simulink model "COSTEP_Exergy"  (R2024b)
settings: Solver=FixedStepAuto  StartTime=0.0  StopTime=25  FixedStep=1/3600  RelTol=1e-3
model workspace (MAT data in the model file):
  AD : Simulink.Parameter (value not decoded)
  AG : Simulink.Parameter (value not decoded)
  AH : Simulink.Parameter (value not decoded)
  AV : Simulink.Parameter (value not decoded)
  AVP : Simulink.Parameter (value not decoded)
  BCHL : Simulink.Parameter (value not decoded)
  BCHV : Simulink.Parameter (value not decoded)
  BD : Simulink.Parameter (value not decoded)
  BDIST : Simulink.Parameter (value not decoded)
  BG : Simulink.Parameter (value not decoded)
  BH : Simulink.Parameter (value not decoded)
  BVP : Simulink.Parameter (value not decoded)
  CD : Simulink.Parameter (value not decoded)
  CDIST : Simulink.Parameter (value not decoded)
  CG : Simulink.Parameter (value not decoded)
  CH : Simulink.Parameter (value not decoded)
  CVP : Simulink.Parameter (value not decoded)
  DDIST : Simulink.Parameter (value not decoded)
  DIST_CONST : Simulink.Parameter (value not decoded)
  ISV : Simulink.Parameter (value not decoded)
  TLAST : Simulink.Parameter (value not decoded)
  TNEXT : Simulink.Parameter (value not decoded)
  XMW : Simulink.Parameter (value not decoded)
  XNS : Simulink.Parameter (value not decoded)
  XNS2 : Simulink.Parameter (value not decoded)
  XNS3 : Simulink.Parameter (value not decoded)
  XNSADD : Simulink.Parameter (value not decoded)
  XNSE : Simulink.Parameter (value not decoded)
symbols that are objects in the model workspace (value not decoded): AD, AG, AH, AV, AVP, BD, BG, BH, BVP, CD, CG, CH, CVP, XMW, XNS, XNS2, XNS3, XNSE
undefined symbols (not defined in the file or in its folder): magnitude, msgbox, SETPT, XMEAS, XMV
libraries: mylib x403, dspindex x31
(part 12 of 13)

== system COSTEP_Exergy/Stream Measurements/Subsystem6/E feed stream/Composition measurement mol%/Subsystem/Subsystem ==
  XST : Inport
  Constant : Constant  Value=100
  Multiport Selector : dspindex/Multiport Selector  rowsOrCols=Rows  idxCellArray={ 5,6}  idxErrMode=Clip Index
  Product : Product
  Product1 : Product
  "XCMPE " : Outport  VectorParamsAs1DForOutWhenUnconnected=off
  "XCMPF " : Outport  Port=2  VectorParamsAs1DForOutWhenUnconnected=off
  wires:
  Multiport Selector/1 -> Product/1
  Constant/1 -> Product/2, Product1/2
  XST/1 -> Multiport Selector/1
  Multiport Selector/2 -> Product1/1
  Product/1 -> "XCMPE "/1
  Product1/1 -> "XCMPF "/1

== system COSTEP_Exergy/Stream Measurements/Subsystem6/Product stream/Composition measurement mol%/Subsystem/Subsystem ==
  XST : Inport
  Constant : Constant  Value=100
  Multiport Selector : dspindex/Multiport Selector  rowsOrCols=Rows  idxCellArray={ 1,2,3}  idxErrMode=Clip Index
  Product : Product
  Product1 : Product
  Product2 : Product
  XCMPA : Outport  VectorParamsAs1DForOutWhenUnconnected=off
  XCMPB : Outport  Port=2  VectorParamsAs1DForOutWhenUnconnected=off
  XCMPC : Outport  Port=3  VectorParamsAs1DForOutWhenUnconnected=off
  wires:
  Multiport Selector/1 -> Product/1
  Multiport Selector/3 -> Product2/1
  Constant/1 -> Product2/2, Product/2, Product1/2
  XST/1 -> Multiport Selector/1
  Multiport Selector/2 -> Product1/1
  Product/1 -> XCMPA/1
  Product1/1 -> XCMPB/1
  Product2/1 -> XCMPC/1

== system COSTEP_Exergy/Stream Measurements/Subsystem6/Product stream/Composition measurement mol%/Subsystem1/Subsystem ==
  XST : Inport
  Constant : Constant  Value=100
  Multiport Selector : dspindex/Multiport Selector  rowsOrCols=Rows  idxCellArray={4,5,6,7,8}  idxErrMode=Clip Index
  "XCMPD " : Product
  XCMPE : Product
  XCMPF : Product
  "XCMPG " : Product
  XCMPH : Product
  XCMPD : Outport  VectorParamsAs1DForOutWhenUnconnected=off
  "XCMPE " : Outport  Port=2  VectorParamsAs1DForOutWhenUnconnected=off
  "XCMPF " : Outport  Port=3  VectorParamsAs1DForOutWhenUnconnected=off
  XCMPG : Outport  Port=4  VectorParamsAs1DForOutWhenUnconnected=off
  "XCMPH " : Outport  Port=5  VectorParamsAs1DForOutWhenUnconnected=off
  wires:
  Constant/1 -> XCMPE/2, "XCMPG "/2, XCMPH/2, XCMPF/2, "XCMPD "/2
  Multiport Selector/1 -> "XCMPD "/1
  "XCMPD "/1 -> XCMPD/1  "XCMPD"
  Multiport Selector/5 -> XCMPH/1
  XCMPF/1 -> "XCMPF "/1  "XCMPF"
  XST/1 -> Multiport Selector/1
  Multiport Selector/4 -> "XCMPG "/1
  Multiport Selector/2 -> XCMPE/1
  Multiport Selector/3 -> XCMPF/1
  XCMPE/1 -> "XCMPE "/1  "XCMPE"
  XCMPH/1 -> "XCMPH "/1  "XCMPH"
  "XCMPG "/1 -> XCMPG/1  "XCMPG"

== system COSTEP_Exergy/Stream Measurements/Subsystem6/Reactor feed stream/Composition measurement mol%/Subsystem/Subsystem ==
  XST : Inport
  Constant : Constant  Value=100
  Multiport Selector : dspindex/Multiport Selector  rowsOrCols=Rows  idxCellArray={7,8}  idxErrMode=Clip Index
  Product6 : Product
  Product7 : Product
  XCMPG : Outport  VectorParamsAs1DForOutWhenUnconnected=off
  "XCMPH " : Outport  Port=2  VectorParamsAs1DForOutWhenUnconnected=off
  wires:
  Multiport Selector/2 -> Product7/1
  Multiport Selector/1 -> Product6/1
  Constant/1 -> Product6/2, Product7/2
  XST/1 -> Multiport Selector/1
  Product6/1 -> XCMPG/1
  Product7/1 -> "XCMPH "/1

== system COSTEP_Exergy/Stream Measurements/Subsystem6/Reactor product stream/Composition measurement mol%/Subsystem/Subsystem ==
  XST : Inport
  Constant : Constant  Value=100
  Multiport Selector : dspindex/Multiport Selector  rowsOrCols=Rows  idxCellArray={ 1,2,3,4,5,6,7,8}  idxErrMode=Clip Index
  Product{,1..7} (8 alike) : Product
  XCMPA : Outport  VectorParamsAs1DForOutWhenUnconnected=off
  XCMPB : Outport  Port=2  VectorParamsAs1DForOutWhenUnconnected=off
  XCMPC : Outport  Port=3  VectorParamsAs1DForOutWhenUnconnected=off
  XCMPD : Outport  Port=4  VectorParamsAs1DForOutWhenUnconnected=off
  "XCMPE " : Outport  Port=5  VectorParamsAs1DForOutWhenUnconnected=off
  "XCMPF " : Outport  Port=6  VectorParamsAs1DForOutWhenUnconnected=off
  XCMPG : Outport  Port=7  VectorParamsAs1DForOutWhenUnconnected=off
  "XCMPH " : Outport  Port=8  VectorParamsAs1DForOutWhenUnconnected=off
  wires:
  Multiport Selector/6 -> Product5/1
  Multiport Selector/8 -> Product7/1
  Multiport Selector/5 -> Product4/1
  Multiport Selector/7 -> Product6/1
  Multiport Selector/1 -> Product/1
  Multiport Selector/3 -> Product2/1
  Constant/1 -> Product/2, Product1/2, Product2/2, Product3/2, Product4/2, Product5/2, Product7/2, Product6/2
  Multiport Selector/4 -> Product3/1
  XST/1 -> Multiport Selector/1
  Multiport Selector/2 -> Product1/1
  Product/1 -> XCMPA/1
  Product1/1 -> XCMPB/1
  Product2/1 -> XCMPC/1
  Product3/1 -> XCMPD/1
  Product4/1 -> "XCMPE "/1
  Product5/1 -> "XCMPF "/1
  Product6/1 -> XCMPG/1
  Product7/1 -> "XCMPH "/1

== system COSTEP_Exergy/Stream Measurements/Subsystem6/Separator product stream/Composition measurement mol%/Subsystem/Subsystem ==
  XST : Inport
  Constant : Constant  Value=100
  Multiport Selector : dspindex/Multiport Selector  rowsOrCols=Rows  idxCellArray={ 1,2,3,4,5,6,7,8}  idxErrMode=Clip Index
  Product{,1..7} (8 alike) : Product
  XCMPA : Outport  VectorParamsAs1DForOutWhenUnconnected=off
  XCMPB : Outport  Port=2  VectorParamsAs1DForOutWhenUnconnected=off
  XCMPC : Outport  Port=3  VectorParamsAs1DForOutWhenUnconnected=off
  XCMPD : Outport  Port=4  VectorParamsAs1DForOutWhenUnconnected=off
  "XCMPE " : Outport  Port=5  VectorParamsAs1DForOutWhenUnconnected=off
  "XCMPF " : Outport  Port=6  VectorParamsAs1DForOutWhenUnconnected=off
  XCMPG : Outport  Port=7  VectorParamsAs1DForOutWhenUnconnected=off
  "XCMPH " : Outport  Port=8  VectorParamsAs1DForOutWhenUnconnected=off
  wires:
  Multiport Selector/6 -> Product5/1
  Multiport Selector/8 -> Product7/1
  Multiport Selector/5 -> Product4/1
  Multiport Selector/7 -> Product6/1
  Multiport Selector/1 -> Product/1
  Multiport Selector/3 -> Product2/1
  Constant/1 -> Product/2, Product1/2, Product2/2, Product3/2, Product4/2, Product5/2, Product7/2, Product6/2
  Multiport Selector/4 -> Product3/1
  XST/1 -> Multiport Selector/1
  Multiport Selector/2 -> Product1/1
  Product/1 -> XCMPA/1
  Product1/1 -> XCMPB/1
  Product2/1 -> XCMPC/1
  Product3/1 -> XCMPD/1
  Product4/1 -> "XCMPE "/1
  Product5/1 -> "XCMPF "/1
  Product6/1 -> XCMPG/1
  Product7/1 -> "XCMPH "/1

== system COSTEP_Exergy/Stream Measurements/Subsystem6/Separator product stream/Flow measurement in kg//h/Subsystem/XMWS Molecular weight of Stream lb//lb-mol ==
  XST : Inport
  Product : Product
  Sum of Elements : Sum  Inputs=+
  "XMW(I) Molecular weight of components lb/lb-mol " : Constant  Value=XMW
  XMWS : Outport  VectorParamsAs1DForOutWhenUnconnected=off
  wires:
  Sum of Elements/1 -> XMWS/1
  Product/1 -> Sum of Elements/1
  XST/1 -> Product/1
  "XMW(I) Molecular weight of components lb/lb-mol "/1 -> Product/2

== system COSTEP_Exergy/Stream Measurements/Subsystem6/Separator product stream/Flow measurement in kg//h/Subsystem1/XMWS Molecular weight of Stream lb//lb-mol ==
  XST : Inport
  Product : Product
  Sum of Elements : Sum  Inputs=+
  "XMW(I) Molecular weight of components lb/lb-mol " : Constant  Value=XMW
  XMWS : Outport  VectorParamsAs1DForOutWhenUnconnected=off
  wires:
  Sum of Elements/1 -> XMWS/1
  Product/1 -> Sum of Elements/1
  XST/1 -> Product/1
  "XMW(I) Molecular weight of components lb/lb-mol "/1 -> Product/2

== system COSTEP_Exergy/Stream Measurements/Subsystem6/Separator recycle stream (after compressor)/Composition measurement mol%/Subsystem/Subsystem ==
  XST : Inport
  Constant : Constant  Value=100
  Multiport Selector : dspindex/Multiport Selector  rowsOrCols=Rows  idxCellArray={ 1,2,3,4,5,6,7,8}  idxErrMode=Clip Index
  Product{,1..7} (8 alike) : Product
  XCMPA : Outport  VectorParamsAs1DForOutWhenUnconnected=off
  XCMPB : Outport  Port=2  VectorParamsAs1DForOutWhenUnconnected=off
  XCMPC : Outport  Port=3  VectorParamsAs1DForOutWhenUnconnected=off
  XCMPD : Outport  Port=4  VectorParamsAs1DForOutWhenUnconnected=off
  "XCMPE " : Outport  Port=5  VectorParamsAs1DForOutWhenUnconnected=off
  "XCMPF " : Outport  Port=6  VectorParamsAs1DForOutWhenUnconnected=off
  XCMPG : Outport  Port=7  VectorParamsAs1DForOutWhenUnconnected=off
  "XCMPH " : Outport  Port=8  VectorParamsAs1DForOutWhenUnconnected=off
  wires:
  Multiport Selector/6 -> Product5/1
  Multiport Selector/8 -> Product7/1
  Multiport Selector/5 -> Product4/1
  Multiport Selector/7 -> Product6/1
  Multiport Selector/1 -> Product/1
  Multiport Selector/3 -> Product2/1
  Constant/1 -> Product/2, Product1/2, Product2/2, Product3/2, Product4/2, Product5/2, Product7/2, Product6/2
  Multiport Selector/4 -> Product3/1
  XST/1 -> Multiport Selector/1
  Multiport Selector/2 -> Product1/1
  Product/1 -> XCMPA/1
  Product1/1 -> XCMPB/1
  Product2/1 -> XCMPC/1
  Product3/1 -> XCMPD/1
  Product4/1 -> "XCMPE "/1
  Product5/1 -> "XCMPF "/1
  Product6/1 -> XCMPG/1
  Product7/1 -> "XCMPH "/1

== system COSTEP_Exergy/Stream Measurements/Subsystem6/Separator recycle stream (before compressor)/Composition measurement mol%/Subsystem/Subsystem ==
  XST : Inport
  Constant : Constant  Value=100
  Multiport Selector : dspindex/Multiport Selector  rowsOrCols=Rows  idxCellArray={ 1,2,3,4,5,6,7,8}  idxErrMode=Clip Index
  Product{,1..7} (8 alike) : Product
  XCMPA : Outport  VectorParamsAs1DForOutWhenUnconnected=off
  XCMPB : Outport  Port=2  VectorParamsAs1DForOutWhenUnconnected=off
  XCMPC : Outport  Port=3  VectorParamsAs1DForOutWhenUnconnected=off
  XCMPD : Outport  Port=4  VectorParamsAs1DForOutWhenUnconnected=off
  "XCMPE " : Outport  Port=5  VectorParamsAs1DForOutWhenUnconnected=off
  "XCMPF " : Outport  Port=6  VectorParamsAs1DForOutWhenUnconnected=off
  XCMPG : Outport  Port=7  VectorParamsAs1DForOutWhenUnconnected=off
  "XCMPH " : Outport  Port=8  VectorParamsAs1DForOutWhenUnconnected=off
  wires:
  Multiport Selector/6 -> Product5/1
  Multiport Selector/8 -> Product7/1
  Multiport Selector/5 -> Product4/1
  Multiport Selector/7 -> Product6/1
  Multiport Selector/1 -> Product/1
  Multiport Selector/3 -> Product2/1
  Constant/1 -> Product/2, Product1/2, Product2/2, Product3/2, Product4/2, Product5/2, Product7/2, Product6/2
  Multiport Selector/4 -> Product3/1
  XST/1 -> Multiport Selector/1
  Multiport Selector/2 -> Product1/1
  Product/1 -> XCMPA/1
  Product1/1 -> XCMPB/1
  Product2/1 -> XCMPC/1
  Product3/1 -> XCMPD/1
  Product4/1 -> "XCMPE "/1
  Product5/1 -> "XCMPF "/1
  Product6/1 -> XCMPG/1
  Product7/1 -> "XCMPH "/1

== system COSTEP_Exergy/Stream Measurements/Subsystem6/Separator underflow stream/Composition measurement mol%/Subsystem/Subsystem ==
  XST : Inport
  Constant : Constant  Value=100
  Multiport Selector : dspindex/Multiport Selector  rowsOrCols=Rows  idxCellArray={ 4,5,6,7,8}  idxErrMode=Clip Index
  Product{3..7} (5 alike) : Product
  XCMPD : Outport  VectorParamsAs1DForOutWhenUnconnected=off
  "XCMPE " : Outport  Port=2  VectorParamsAs1DForOutWhenUnconnected=off
  "XCMPF " : Outport  Port=3  VectorParamsAs1DForOutWhenUnconnected=off
  XCMPG : Outport  Port=4  VectorParamsAs1DForOutWhenUnconnected=off
  "XCMPH " : Outport  Port=5  VectorParamsAs1DForOutWhenUnconnected=off
  wires:
  Constant/1 -> Product3/2, Product4/2, Product5/2, Product7/2, Product6/2
  XST/1 -> Multiport Selector/1
  Product3/1 -> XCMPD/1
  Product4/1 -> "XCMPE "/1
  Product5/1 -> "XCMPF "/1
  Product6/1 -> XCMPG/1
  Product7/1 -> "XCMPH "/1
  Multiport Selector/1 -> Product3/1
  Multiport Selector/2 -> Product4/1
  Multiport Selector/3 -> Product5/1
  Multiport Selector/4 -> Product6/1
  Multiport Selector/5 -> Product7/1

== system COSTEP_Exergy/Stream Measurements/Subsystem6/Stripper recycle stream/Composition measurement mol%/Subsystem/Subsystem ==
  XST : Inport
  Constant : Constant  Value=100
  Multiport Selector : dspindex/Multiport Selector  rowsOrCols=Rows  idxCellArray={ 1,2,3,4,5,6,7,8}  idxErrMode=Clip Index
  Product{,1..7} (8 alike) : Product
  XCMPA : Outport  VectorParamsAs1DForOutWhenUnconnected=off
  XCMPB : Outport  Port=2  VectorParamsAs1DForOutWhenUnconnected=off
  XCMPC : Outport  Port=3  VectorParamsAs1DForOutWhenUnconnected=off
  XCMPD : Outport  Port=4  VectorParamsAs1DForOutWhenUnconnected=off
  "XCMPE " : Outport  Port=5  VectorParamsAs1DForOutWhenUnconnected=off
  "XCMPF " : Outport  Port=6  VectorParamsAs1DForOutWhenUnconnected=off
  XCMPG : Outport  Port=7  VectorParamsAs1DForOutWhenUnconnected=off
  "XCMPH " : Outport  Port=8  VectorParamsAs1DForOutWhenUnconnected=off
  wires:
  Multiport Selector/6 -> Product5/1
  Multiport Selector/8 -> Product7/1
  Multiport Selector/5 -> Product4/1
  Multiport Selector/7 -> Product6/1
  Multiport Selector/1 -> Product/1
  Multiport Selector/3 -> Product2/1
  Constant/1 -> Product/2, Product1/2, Product2/2, Product3/2, Product4/2, Product5/2, Product7/2, Product6/2
  Multiport Selector/4 -> Product3/1
  XST/1 -> Multiport Selector/1
  Multiport Selector/2 -> Product1/1
  Product/1 -> XCMPA/1
  Product1/1 -> XCMPB/1
  Product2/1 -> XCMPC/1
  Product3/1 -> XCMPD/1
  Product4/1 -> "XCMPE "/1
  Product5/1 -> "XCMPF "/1
  Product6/1 -> XCMPG/1
  Product7/1 -> "XCMPH "/1

== system COSTEP_Exergy/Subsystem1/Condenser cooling water/CCin/Subsystem3/Subsystem/Subsystem2 ==
  T1 : Inport
  T0 : Inport  Port=2
  A : Constant  Value=9.069
  Add1 : Sum  Inputs=+-
  Product1 : Product
  AT : Outport
  wires:
  Add1/1 -> Product1/2
  A/1 -> Product1/1
  T0/1 -> Add1/2
  T1/1 -> Add1/1
  Product1/1 -> AT/1

== system COSTEP_Exergy/Subsystem1/Condenser cooling water/CCin/Subsystem3/Subsystem1/Subsystem ==
  T1 : Inport
  T0 : Inport  Port=2
  A : Constant  Value=9.069
  Divide : Product  Inputs=*/
  Math Function : Math  Operator=log  SignedPower=on
  Product1 : Product
  AT : Outport
  wires:
  Product1/1 -> AT/1
  A/1 -> Product1/1
  T1/1 -> Divide/1
  T0/1 -> Divide/2
  Math Function/1 -> Product1/2
  Divide/1 -> Math Function/1

== system COSTEP_Exergy/Subsystem1/Condenser cooling water/CCout/Subsystem3/Subsystem/Subsystem2 ==
  T1 : Inport
  T0 : Inport  Port=2
  A : Constant  Value=9.069
  Add1 : Sum  Inputs=+-
  Product1 : Product
  AT : Outport
  wires:
  Add1/1 -> Product1/2
  A/1 -> Product1/1
  T0/1 -> Add1/2
  T1/1 -> Add1/1
  Product1/1 -> AT/1

== system COSTEP_Exergy/Subsystem1/Condenser cooling water/CCout/Subsystem3/Subsystem1/Subsystem ==
  T1 : Inport
  T0 : Inport  Port=2
  A : Constant  Value=9.069
  Divide : Product  Inputs=*/
  Math Function : Math  Operator=log  SignedPower=on
  Product1 : Product
  AT : Outport
  wires:
  Product1/1 -> AT/1
  A/1 -> Product1/1
  T1/1 -> Divide/1
  T0/1 -> Divide/2
  Math Function/1 -> Product1/2
  Divide/1 -> Math Function/1

== system COSTEP_Exergy/Subsystem1/Reactor cooling water/RCin/Subsystem3/Subsystem/Subsystem2 ==
  T1 : Inport
  T0 : Inport  Port=2
  A : Constant  Value=9.069
  Add1 : Sum  Inputs=+-
  Product1 : Product
  AT : Outport
  wires:
  Add1/1 -> Product1/2
  A/1 -> Product1/1
  T0/1 -> Add1/2
  T1/1 -> Add1/1
  Product1/1 -> AT/1

== system COSTEP_Exergy/Subsystem1/Reactor cooling water/RCin/Subsystem3/Subsystem1/Subsystem ==
  T1 : Inport
  T0 : Inport  Port=2
  A : Constant  Value=9.069
  Divide : Product  Inputs=*/
  Math Function : Math  Operator=log  SignedPower=on
  Product1 : Product
  AT : Outport
  wires:
  Product1/1 -> AT/1
  A/1 -> Product1/1
  T1/1 -> Divide/1
  T0/1 -> Divide/2
  Math Function/1 -> Product1/2
  Divide/1 -> Math Function/1

== system COSTEP_Exergy/Subsystem1/Reactor cooling water/RCout/Subsystem3/Subsystem/Subsystem2 ==
  T1 : Inport
  T0 : Inport  Port=2
  A : Constant  Value=9.069
  Add1 : Sum  Inputs=+-
  Product1 : Product
  AT : Outport
  wires:
  Add1/1 -> Product1/2
  A/1 -> Product1/1
  T0/1 -> Add1/2
  T1/1 -> Add1/1
  Product1/1 -> AT/1

== system COSTEP_Exergy/Subsystem1/Reactor cooling water/RCout/Subsystem3/Subsystem1/Subsystem ==
  T1 : Inport
  T0 : Inport  Port=2
  A : Constant  Value=9.069
  Divide : Product  Inputs=*/
  Math Function : Math  Operator=log  SignedPower=on
  Product1 : Product
  AT : Outport
  wires:
  Product1/1 -> AT/1
  A/1 -> Product1/1
  T1/1 -> Divide/1
  T0/1 -> Divide/2
  Math Function/1 -> Product1/2
  Divide/1 -> Math Function/1

== system COSTEP_Exergy/Control Mode/Braatz/ 10/CONTROL 6/P Control Velocity form/Pressure limits/If Action Subsystem ==
  In1 : Inport
  Action Port : ActionPort  ActionPortLabel=if(u1 >= 2950)
  Out1 : Outport  VectorParamsAs1DForOutWhenUnconnected=off
  wires:
  In1/1 -> Out1/1

== system COSTEP_Exergy/Control Mode/Braatz/ 10/CONTROL 6/P Control Velocity form/Pressure limits/If Action Subsystem1 ==
  In1 : Inport
  Action Port : ActionPort  ActionPortLabel=elseif(u1 <= 2300)
  Out1 : Outport  VectorParamsAs1DForOutWhenUnconnected=off
  wires:
  In1/1 -> Out1/1

== system COSTEP_Exergy/Control Mode/Braatz/ 10/CONTROL 6/P Control Velocity form/Pressure limits/If Action Subsystem2 ==
  In1 : Inport
  Action Port : ActionPort  ActionPortLabel=else
  Out1 : Outport  VectorParamsAs1DForOutWhenUnconnected=off
  wires:
  In1/1 -> Out1/1

== system COSTEP_Exergy/Random number generator/Stream Measurements SMEAS Gas analysis1/If Action Subsystem3/Subsystem/Stream 1/Subsystem/TESUB6 XMNSEA ==
  G : Inport
  Process Noise I=1-12 G New : mylib/Process Noise I=1-12 G New  SystemSampleTime=-1  VariantActivationTime=update diagram  AllowFlexibleInterface=on  Latency=0  AutoFrameSizeCalculation=off
  XNSEA : Constant  Value=0.25
  XMNSEA : Outport  VectorParamsAs1DForOutWhenUnconnected=off
  G_NEW : Outport  Port=2  VectorParamsAs1DForOutWhenUnconnected=off
  wires:
  XNSEA/1 -> Process Noise I=1-12 G New/1
  Process Noise I=1-12 G New/1 -> XMNSEA/1
  G/1 -> Process Noise I=1-12 G New/2
  Process Noise I=1-12 G New/2 -> G_NEW/1

== system COSTEP_Exergy/Random number generator/Stream Measurements SMEAS Gas analysis1/If Action Subsystem3/Subsystem/Stream 1/Subsystem/TESUB6 XMNSEB ==
  G : Inport
  Process Noise I=1-12 G New : mylib/Process Noise I=1-12 G New  SystemSampleTime=-1  VariantActivationTime=update diagram  AllowFlexibleInterface=on  Latency=0  AutoFrameSizeCalculation=off
  XNSEB : Constant  Value=0.1
  XMNSEB : Outport  VectorParamsAs1DForOutWhenUnconnected=off
  G_NEW : Outport  Port=2  VectorParamsAs1DForOutWhenUnconnected=off
  wires:
  XNSEB/1 -> Process Noise I=1-12 G New/1
  Process Noise I=1-12 G New/1 -> XMNSEB/1
  G/1 -> Process Noise I=1-12 G New/2
  Process Noise I=1-12 G New/2 -> G_NEW/1

== system COSTEP_Exergy/Random number generator/Stream Measurements SMEAS Gas analysis1/If Action Subsystem3/Subsystem/Stream 1/Subsystem/TESUB6 XMNSEC ==
  G : Inport
  Process Noise I=1-12 G New : mylib/Process Noise I=1-12 G New  SystemSampleTime=-1  VariantActivationTime=update diagram  AllowFlexibleInterface=on  Latency=0  AutoFrameSizeCalculation=off
  XNSEC : Constant  Value=0.25
  XMNSEC : Outport  VectorParamsAs1DForOutWhenUnconnected=off
  G_NEW : Outport  Port=2  VectorParamsAs1DForOutWhenUnconnected=off
  wires:
  XNSEC/1 -> Process Noise I=1-12 G New/1
  Process Noise I=1-12 G New/1 -> XMNSEC/1
  G/1 -> Process Noise I=1-12 G New/2
  Process Noise I=1-12 G New/2 -> G_NEW/1

== system COSTEP_Exergy/Random number generator/Stream Measurements SMEAS Gas analysis1/If Action Subsystem3/Subsystem/Stream 1/Subsystem/TESUB6 XMNSED ==
  G : Inport
  Process Noise I=1-12 G New : mylib/Process Noise I=1-12 G New  SystemSampleTime=-1  VariantActivationTime=update diagram  AllowFlexibleInterface=on  Latency=0  AutoFrameSizeCalculation=off
  XNSED : Constant  Value=0.1
  XMNSED : Outport  VectorParamsAs1DForOutWhenUnconnected=off
  G_NEW : Outport  Port=2  VectorParamsAs1DForOutWhenUnconnected=off
  wires:
  XNSED/1 -> Process Noise I=1-12 G New/1
  Process Noise I=1-12 G New/1 -> XMNSED/1
  G/1 -> Process Noise I=1-12 G New/2
  Process Noise I=1-12 G New/2 -> G_NEW/1

== system COSTEP_Exergy/Random number generator/Stream Measurements SMEAS Gas analysis1/If Action Subsystem3/Subsystem/Stream 1/Subsystem/TESUB6 XMNSEE ==
  G : Inport
  Process Noise I=1-12 G New : mylib/Process Noise I=1-12 G New  SystemSampleTime=-1  VariantActivationTime=update diagram  AllowFlexibleInterface=on  Latency=0  AutoFrameSizeCalculation=off
  XNSEE : Constant  Value=0.25
  XMNSEE : Outport  VectorParamsAs1DForOutWhenUnconnected=off
  G_NEW : Outport  Port=2  VectorParamsAs1DForOutWhenUnconnected=off
  wires:
  XNSEE/1 -> Process Noise I=1-12 G New/1
  Process Noise I=1-12 G New/1 -> XMNSEE/1
  G/1 -> Process Noise I=1-12 G New/2
  Process Noise I=1-12 G New/2 -> G_NEW/1

== system COSTEP_Exergy/Random number generator/Stream Measurements SMEAS Gas analysis1/If Action Subsystem3/Subsystem/Stream 1/Subsystem/TESUB6 XMNSEF ==
  G : Inport
  Process Noise I=1-12 G New : mylib/Process Noise I=1-12 G New  SystemSampleTime=-1  VariantActivationTime=update diagram  AllowFlexibleInterface=on  Latency=0  AutoFrameSizeCalculation=off
  XNSEF : Constant  Value=0.025
  XMNSEF : Outport  VectorParamsAs1DForOutWhenUnconnected=off
  G_NEW : Outport  Port=2  VectorParamsAs1DForOutWhenUnconnected=off
  wires:
  XNSEF/1 -> Process Noise I=1-12 G New/1
  Process Noise I=1-12 G New/1 -> XMNSEF/1
  G/1 -> Process Noise I=1-12 G New/2
  Process Noise I=1-12 G New/2 -> G_NEW/1

== system COSTEP_Exergy/Random number generator/Stream Measurements SMEAS Gas analysis1/If Action Subsystem3/Subsystem/Stream 1/Subsystem/TESUB6 XMNSEG ==
  G : Inport
  Process Noise I=1-12 G New : mylib/Process Noise I=1-12 G New  SystemSampleTime=-1  VariantActivationTime=update diagram  AllowFlexibleInterface=on  Latency=0  AutoFrameSizeCalculation=off
  XNSEG : Constant  Value=0.05
  XMNSEG : Outport  VectorParamsAs1DForOutWhenUnconnected=off
  G_NEW : Outport  Port=2  VectorParamsAs1DForOutWhenUnconnected=off
  wires:
  XNSEG/1 -> Process Noise I=1-12 G New/1
  Process Noise I=1-12 G New/1 -> XMNSEG/1
  G/1 -> Process Noise I=1-12 G New/2
  Process Noise I=1-12 G New/2 -> G_NEW/1

== system COSTEP_Exergy/Random number generator/Stream Measurements SMEAS Gas analysis1/If Action Subsystem3/Subsystem/Stream 1/Subsystem/TESUB6 XMNSEH ==
  G : Inport
  Process Noise I=1-12 G New : mylib/Process Noise I=1-12 G New  SystemSampleTime=-1  VariantActivationTime=update diagram  AllowFlexibleInterface=on  Latency=0  AutoFrameSizeCalculation=off
  XNSEH : Constant  Value=0.05
  XMNSEH : Outport  VectorParamsAs1DForOutWhenUnconnected=off
  G_NEW : Outport  Port=2  VectorParamsAs1DForOutWhenUnconnected=off
  wires:
  XNSEH/1 -> Process Noise I=1-12 G New/1
  Process Noise I=1-12 G New/1 -> XMNSEH/1
  G/1 -> Process Noise I=1-12 G New/2
  Process Noise I=1-12 G New/2 -> G_NEW/1

== system COSTEP_Exergy/Random number generator/Stream Measurements SMEAS Gas analysis1/If Action Subsystem3/Subsystem/Stream 13/Subsystem/TESUB6 XMNSEA ==
  G : Inport
  Process Noise I=1-12 G New : mylib/Process Noise I=1-12 G New  SystemSampleTime=-1  VariantActivationTime=update diagram  AllowFlexibleInterface=on  Latency=0  AutoFrameSizeCalculation=off
  XNSEA : Constant  Value=0.25
  XMNSEA : Outport  VectorParamsAs1DForOutWhenUnconnected=off
  G_NEW : Outport  Port=2  VectorParamsAs1DForOutWhenUnconnected=off
  wires:
  XNSEA/1 -> Process Noise I=1-12 G New/1
  Process Noise I=1-12 G New/1 -> XMNSEA/1
  G/1 -> Process Noise I=1-12 G New/2
  Process Noise I=1-12 G New/2 -> G_NEW/1

== system COSTEP_Exergy/Random number generator/Stream Measurements SMEAS Gas analysis1/If Action Subsystem3/Subsystem/Stream 13/Subsystem/TESUB6 XMNSEB ==
  G : Inport
  Process Noise I=1-12 G New : mylib/Process Noise I=1-12 G New  SystemSampleTime=-1  VariantActivationTime=update diagram  AllowFlexibleInterface=on  Latency=0  AutoFrameSizeCalculation=off
  XNSEB : Constant  Value=0.1
  XMNSEB : Outport  VectorParamsAs1DForOutWhenUnconnected=off
  G_NEW : Outport  Port=2  VectorParamsAs1DForOutWhenUnconnected=off
  wires:
  XNSEB/1 -> Process Noise I=1-12 G New/1
  Process Noise I=1-12 G New/1 -> XMNSEB/1
  G/1 -> Process Noise I=1-12 G New/2
  Process Noise I=1-12 G New/2 -> G_NEW/1

== system COSTEP_Exergy/Random number generator/Stream Measurements SMEAS Gas analysis1/If Action Subsystem3/Subsystem/Stream 13/Subsystem/TESUB6 XMNSEC ==
  G : Inport
  Process Noise I=1-12 G New : mylib/Process Noise I=1-12 G New  SystemSampleTime=-1  VariantActivationTime=update diagram  AllowFlexibleInterface=on  Latency=0  AutoFrameSizeCalculation=off
  XNSEC : Constant  Value=0.25
  XMNSEC : Outport  VectorParamsAs1DForOutWhenUnconnected=off
  G_NEW : Outport  Port=2  VectorParamsAs1DForOutWhenUnconnected=off
  wires:
  XNSEC/1 -> Process Noise I=1-12 G New/1
  Process Noise I=1-12 G New/1 -> XMNSEC/1
  G/1 -> Process Noise I=1-12 G New/2
  Process Noise I=1-12 G New/2 -> G_NEW/1

== system COSTEP_Exergy/Random number generator/Stream Measurements SMEAS Gas analysis1/If Action Subsystem3/Subsystem/Stream 13/Subsystem/TESUB6 XMNSED ==
  G : Inport
  Process Noise I=1-12 G New : mylib/Process Noise I=1-12 G New  SystemSampleTime=-1  VariantActivationTime=update diagram  AllowFlexibleInterface=on  Latency=0  AutoFrameSizeCalculation=off
  XNSED : Constant  Value=0.1
  XMNSED : Outport  VectorParamsAs1DForOutWhenUnconnected=off
  G_NEW : Outport  Port=2  VectorParamsAs1DForOutWhenUnconnected=off
  wires:
  XNSED/1 -> Process Noise I=1-12 G New/1
  Process Noise I=1-12 G New/1 -> XMNSED/1
  G/1 -> Process Noise I=1-12 G New/2
  Process Noise I=1-12 G New/2 -> G_NEW/1

== system COSTEP_Exergy/Random number generator/Stream Measurements SMEAS Gas analysis1/If Action Subsystem3/Subsystem/Stream 13/Subsystem/TESUB6 XMNSEE ==
  G : Inport
  Process Noise I=1-12 G New : mylib/Process Noise I=1-12 G New  SystemSampleTime=-1  VariantActivationTime=update diagram  AllowFlexibleInterface=on  Latency=0  AutoFrameSizeCalculation=off
  XNSEE : Constant  Value=0.25
  XMNSEE : Outport  VectorParamsAs1DForOutWhenUnconnected=off
  G_NEW : Outport  Port=2  VectorParamsAs1DForOutWhenUnconnected=off
  wires:
  XNSEE/1 -> Process Noise I=1-12 G New/1
  Process Noise I=1-12 G New/1 -> XMNSEE/1
  G/1 -> Process Noise I=1-12 G New/2
  Process Noise I=1-12 G New/2 -> G_NEW/1

== system COSTEP_Exergy/Random number generator/Stream Measurements SMEAS Gas analysis1/If Action Subsystem3/Subsystem/Stream 13/Subsystem/TESUB6 XMNSEF ==
  G : Inport
  Process Noise I=1-12 G New : mylib/Process Noise I=1-12 G New  SystemSampleTime=-1  VariantActivationTime=update diagram  AllowFlexibleInterface=on  Latency=0  AutoFrameSizeCalculation=off
  XNSEF : Constant  Value=0.025
  XMNSEF : Outport  VectorParamsAs1DForOutWhenUnconnected=off
  G_NEW : Outport  Port=2  VectorParamsAs1DForOutWhenUnconnected=off
  wires:
  XNSEF/1 -> Process Noise I=1-12 G New/1
  Process Noise I=1-12 G New/1 -> XMNSEF/1
  G/1 -> Process Noise I=1-12 G New/2
  Process Noise I=1-12 G New/2 -> G_NEW/1

== system COSTEP_Exergy/Random number generator/Stream Measurements SMEAS Gas analysis1/If Action Subsystem3/Subsystem/Stream 13/Subsystem/TESUB6 XMNSEG ==
  G : Inport
  Process Noise I=1-12 G New : mylib/Process Noise I=1-12 G New  SystemSampleTime=-1  VariantActivationTime=update diagram  AllowFlexibleInterface=on  Latency=0  AutoFrameSizeCalculation=off
  XNSEG : Constant  Value=0.05
  XMNSEG : Outport  VectorParamsAs1DForOutWhenUnconnected=off
  G_NEW : Outport  Port=2  VectorParamsAs1DForOutWhenUnconnected=off
  wires:
  XNSEG/1 -> Process Noise I=1-12 G New/1
  Process Noise I=1-12 G New/1 -> XMNSEG/1
  G/1 -> Process Noise I=1-12 G New/2
  Process Noise I=1-12 G New/2 -> G_NEW/1

== system COSTEP_Exergy/Random number generator/Stream Measurements SMEAS Gas analysis1/If Action Subsystem3/Subsystem/Stream 13/Subsystem/TESUB6 XMNSEH ==
  G : Inport
  Process Noise I=1-12 G New : mylib/Process Noise I=1-12 G New  SystemSampleTime=-1  VariantActivationTime=update diagram  AllowFlexibleInterface=on  Latency=0  AutoFrameSizeCalculation=off
  XNSEH : Constant  Value=0.05
  XMNSEH : Outport  VectorParamsAs1DForOutWhenUnconnected=off
  G_NEW : Outport  Port=2  VectorParamsAs1DForOutWhenUnconnected=off
  wires:
  XNSEH/1 -> Process Noise I=1-12 G New/1
  Process Noise I=1-12 G New/1 -> XMNSEH/1
  G/1 -> Process Noise I=1-12 G New/2
  Process Noise I=1-12 G New/2 -> G_NEW/1

== system COSTEP_Exergy/Random number generator/Stream Measurements SMEAS Gas analysis1/If Action Subsystem3/Subsystem/Stream 2/Subsystem/TESUB6 XMNSEA ==
  G : Inport
  Process Noise I=1-12 G New : mylib/Process Noise I=1-12 G New  SystemSampleTime=-1  VariantActivationTime=update diagram  AllowFlexibleInterface=on  Latency=0  AutoFrameSizeCalculation=off
  XNSEA : Constant  Value=0.25
  XMNSEA : Outport  VectorParamsAs1DForOutWhenUnconnected=off
  G_NEW : Outport  Port=2  VectorParamsAs1DForOutWhenUnconnected=off
  wires:
  XNSEA/1 -> Process Noise I=1-12 G New/1
  Process Noise I=1-12 G New/1 -> XMNSEA/1
  G/1 -> Process Noise I=1-12 G New/2
  Process Noise I=1-12 G New/2 -> G_NEW/1

== system COSTEP_Exergy/Random number generator/Stream Measurements SMEAS Gas analysis1/If Action Subsystem3/Subsystem/Stream 2/Subsystem/TESUB6 XMNSEB ==
  G : Inport
  Process Noise I=1-12 G New : mylib/Process Noise I=1-12 G New  SystemSampleTime=-1  VariantActivationTime=update diagram  AllowFlexibleInterface=on  Latency=0  AutoFrameSizeCalculation=off
  XNSEB : Constant  Value=0.1
  XMNSEB : Outport  VectorParamsAs1DForOutWhenUnconnected=off
  G_NEW : Outport  Port=2  VectorParamsAs1DForOutWhenUnconnected=off
  wires:
  XNSEB/1 -> Process Noise I=1-12 G New/1
  Process Noise I=1-12 G New/1 -> XMNSEB/1
  G/1 -> Process Noise I=1-12 G New/2
  Process Noise I=1-12 G New/2 -> G_NEW/1

== system COSTEP_Exergy/Random number generator/Stream Measurements SMEAS Gas analysis1/If Action Subsystem3/Subsystem/Stream 2/Subsystem/TESUB6 XMNSEC ==
  G : Inport
  Process Noise I=1-12 G New : mylib/Process Noise I=1-12 G New  SystemSampleTime=-1  VariantActivationTime=update diagram  AllowFlexibleInterface=on  Latency=0  AutoFrameSizeCalculation=off
  XNSEC : Constant  Value=0.25
  XMNSEC : Outport  VectorParamsAs1DForOutWhenUnconnected=off
  G_NEW : Outport  Port=2  VectorParamsAs1DForOutWhenUnconnected=off
  wires:
  XNSEC/1 -> Process Noise I=1-12 G New/1
  Process Noise I=1-12 G New/1 -> XMNSEC/1
  G/1 -> Process Noise I=1-12 G New/2
  Process Noise I=1-12 G New/2 -> G_NEW/1

== system COSTEP_Exergy/Random number generator/Stream Measurements SMEAS Gas analysis1/If Action Subsystem3/Subsystem/Stream 2/Subsystem/TESUB6 XMNSED ==
  G : Inport
  Process Noise I=1-12 G New : mylib/Process Noise I=1-12 G New  SystemSampleTime=-1  VariantActivationTime=update diagram  AllowFlexibleInterface=on  Latency=0  AutoFrameSizeCalculation=off
  XNSED : Constant  Value=0.1
  XMNSED : Outport  VectorParamsAs1DForOutWhenUnconnected=off
  G_NEW : Outport  Port=2  VectorParamsAs1DForOutWhenUnconnected=off
  wires:
  XNSED/1 -> Process Noise I=1-12 G New/1
  Process Noise I=1-12 G New/1 -> XMNSED/1
  G/1 -> Process Noise I=1-12 G New/2
  Process Noise I=1-12 G New/2 -> G_NEW/1

== system COSTEP_Exergy/Random number generator/Stream Measurements SMEAS Gas analysis1/If Action Subsystem3/Subsystem/Stream 2/Subsystem/TESUB6 XMNSEE ==
  G : Inport
  Process Noise I=1-12 G New : mylib/Process Noise I=1-12 G New  SystemSampleTime=-1  VariantActivationTime=update diagram  AllowFlexibleInterface=on  Latency=0  AutoFrameSizeCalculation=off
  XNSEE : Constant  Value=0.25
  XMNSEE : Outport  VectorParamsAs1DForOutWhenUnconnected=off
  G_NEW : Outport  Port=2  VectorParamsAs1DForOutWhenUnconnected=off
  wires:
  XNSEE/1 -> Process Noise I=1-12 G New/1
  Process Noise I=1-12 G New/1 -> XMNSEE/1
  G/1 -> Process Noise I=1-12 G New/2
  Process Noise I=1-12 G New/2 -> G_NEW/1

== system COSTEP_Exergy/Random number generator/Stream Measurements SMEAS Gas analysis1/If Action Subsystem3/Subsystem/Stream 2/Subsystem/TESUB6 XMNSEF ==
  G : Inport
  Process Noise I=1-12 G New : mylib/Process Noise I=1-12 G New  SystemSampleTime=-1  VariantActivationTime=update diagram  AllowFlexibleInterface=on  Latency=0  AutoFrameSizeCalculation=off
  XNSEF : Constant  Value=0.025
  XMNSEF : Outport  VectorParamsAs1DForOutWhenUnconnected=off
  G_NEW : Outport  Port=2  VectorParamsAs1DForOutWhenUnconnected=off
  wires:
  XNSEF/1 -> Process Noise I=1-12 G New/1
  Process Noise I=1-12 G New/1 -> XMNSEF/1
  G/1 -> Process Noise I=1-12 G New/2
  Process Noise I=1-12 G New/2 -> G_NEW/1

== system COSTEP_Exergy/Random number generator/Stream Measurements SMEAS Gas analysis1/If Action Subsystem3/Subsystem/Stream 2/Subsystem/TESUB6 XMNSEG ==
  G : Inport
  Process Noise I=1-12 G New : mylib/Process Noise I=1-12 G New  SystemSampleTime=-1  VariantActivationTime=update diagram  AllowFlexibleInterface=on  Latency=0  AutoFrameSizeCalculation=off
  XNSEG : Constant  Value=0.05
  XMNSEG : Outport  VectorParamsAs1DForOutWhenUnconnected=off
  G_NEW : Outport  Port=2  VectorParamsAs1DForOutWhenUnconnected=off
  wires:
  XNSEG/1 -> Process Noise I=1-12 G New/1
  Process Noise I=1-12 G New/1 -> XMNSEG/1
  G/1 -> Process Noise I=1-12 G New/2
  Process Noise I=1-12 G New/2 -> G_NEW/1

== system COSTEP_Exergy/Random number generator/Stream Measurements SMEAS Gas analysis1/If Action Subsystem3/Subsystem/Stream 2/Subsystem/TESUB6 XMNSEH ==
  G : Inport
  Process Noise I=1-12 G New : mylib/Process Noise I=1-12 G New  SystemSampleTime=-1  VariantActivationTime=update diagram  AllowFlexibleInterface=on  Latency=0  AutoFrameSizeCalculation=off
  XNSEH : Constant  Value=0.05
  XMNSEH : Outport  VectorParamsAs1DForOutWhenUnconnected=off
  G_NEW : Outport  Port=2  VectorParamsAs1DForOutWhenUnconnected=off
  wires:
  XNSEH/1 -> Process Noise I=1-12 G New/1
  Process Noise I=1-12 G New/1 -> XMNSEH/1
  G/1 -> Process Noise I=1-12 G New/2
  Process Noise I=1-12 G New/2 -> G_NEW/1

== system COSTEP_Exergy/Random number generator/Stream Measurements SMEAS Gas analysis1/If Action Subsystem3/Subsystem/Stream 3/Subsystem/TESUB6 XMNSEA ==
  G : Inport
  Process Noise I=1-12 G New : mylib/Process Noise I=1-12 G New  SystemSampleTime=-1  VariantActivationTime=update diagram  AllowFlexibleInterface=on  Latency=0  AutoFrameSizeCalculation=off
  XNSEA : Constant  Value=0.25
  XMNSEA : Outport  VectorParamsAs1DForOutWhenUnconnected=off
  G_NEW : Outport  Port=2  VectorParamsAs1DForOutWhenUnconnected=off
  wires:
  XNSEA/1 -> Process Noise I=1-12 G New/1
  Process Noise I=1-12 G New/1 -> XMNSEA/1
  G/1 -> Process Noise I=1-12 G New/2
  Process Noise I=1-12 G New/2 -> G_NEW/1

== system COSTEP_Exergy/Random number generator/Stream Measurements SMEAS Gas analysis1/If Action Subsystem3/Subsystem/Stream 3/Subsystem/TESUB6 XMNSEB ==
  G : Inport
  Process Noise I=1-12 G New : mylib/Process Noise I=1-12 G New  SystemSampleTime=-1  VariantActivationTime=update diagram  AllowFlexibleInterface=on  Latency=0  AutoFrameSizeCalculation=off
  XNSEB : Constant  Value=0.1
  XMNSEB : Outport  VectorParamsAs1DForOutWhenUnconnected=off
  G_NEW : Outport  Port=2  VectorParamsAs1DForOutWhenUnconnected=off
  wires:
  XNSEB/1 -> Process Noise I=1-12 G New/1
  Process Noise I=1-12 G New/1 -> XMNSEB/1
  G/1 -> Process Noise I=1-12 G New/2
  Process Noise I=1-12 G New/2 -> G_NEW/1

== system COSTEP_Exergy/Random number generator/Stream Measurements SMEAS Gas analysis1/If Action Subsystem3/Subsystem/Stream 3/Subsystem/TESUB6 XMNSEC ==
  G : Inport
  Process Noise I=1-12 G New : mylib/Process Noise I=1-12 G New  SystemSampleTime=-1  VariantActivationTime=update diagram  AllowFlexibleInterface=on  Latency=0  AutoFrameSizeCalculation=off
  XNSEC : Constant  Value=0.25
  XMNSEC : Outport  VectorParamsAs1DForOutWhenUnconnected=off
  G_NEW : Outport  Port=2  VectorParamsAs1DForOutWhenUnconnected=off
  wires:
  XNSEC/1 -> Process Noise I=1-12 G New/1
  Process Noise I=1-12 G New/1 -> XMNSEC/1
  G/1 -> Process Noise I=1-12 G New/2
  Process Noise I=1-12 G New/2 -> G_NEW/1

== system COSTEP_Exergy/Random number generator/Stream Measurements SMEAS Gas analysis1/If Action Subsystem3/Subsystem/Stream 3/Subsystem/TESUB6 XMNSED ==
  G : Inport
  Process Noise I=1-12 G New : mylib/Process Noise I=1-12 G New  SystemSampleTime=-1  VariantActivationTime=update diagram  AllowFlexibleInterface=on  Latency=0  AutoFrameSizeCalculation=off
  XNSED : Constant  Value=0.1
  XMNSED : Outport  VectorParamsAs1DForOutWhenUnconnected=off
  G_NEW : Outport  Port=2  VectorParamsAs1DForOutWhenUnconnected=off
  wires:
  XNSED/1 -> Process Noise I=1-12 G New/1
  Process Noise I=1-12 G New/1 -> XMNSED/1
  G/1 -> Process Noise I=1-12 G New/2
  Process Noise I=1-12 G New/2 -> G_NEW/1

== system COSTEP_Exergy/Random number generator/Stream Measurements SMEAS Gas analysis1/If Action Subsystem3/Subsystem/Stream 3/Subsystem/TESUB6 XMNSEE ==
  G : Inport
  Process Noise I=1-12 G New : mylib/Process Noise I=1-12 G New  SystemSampleTime=-1  VariantActivationTime=update diagram  AllowFlexibleInterface=on  Latency=0  AutoFrameSizeCalculation=off
  XNSEE : Constant  Value=0.25
  XMNSEE : Outport  VectorParamsAs1DForOutWhenUnconnected=off
  G_NEW : Outport  Port=2  VectorParamsAs1DForOutWhenUnconnected=off
  wires:
  XNSEE/1 -> Process Noise I=1-12 G New/1
  Process Noise I=1-12 G New/1 -> XMNSEE/1
  G/1 -> Process Noise I=1-12 G New/2
  Process Noise I=1-12 G New/2 -> G_NEW/1

== system COSTEP_Exergy/Random number generator/Stream Measurements SMEAS Gas analysis1/If Action Subsystem3/Subsystem/Stream 3/Subsystem/TESUB6 XMNSEF ==
  G : Inport
  Process Noise I=1-12 G New : mylib/Process Noise I=1-12 G New  SystemSampleTime=-1  VariantActivationTime=update diagram  AllowFlexibleInterface=on  Latency=0  AutoFrameSizeCalculation=off
  XNSEF : Constant  Value=0.025
  XMNSEF : Outport  VectorParamsAs1DForOutWhenUnconnected=off
  G_NEW : Outport  Port=2  VectorParamsAs1DForOutWhenUnconnected=off
  wires:
  XNSEF/1 -> Process Noise I=1-12 G New/1
  Process Noise I=1-12 G New/1 -> XMNSEF/1
  G/1 -> Process Noise I=1-12 G New/2
  Process Noise I=1-12 G New/2 -> G_NEW/1

== system COSTEP_Exergy/Random number generator/Stream Measurements SMEAS Gas analysis1/If Action Subsystem3/Subsystem/Stream 3/Subsystem/TESUB6 XMNSEG ==
  G : Inport
  Process Noise I=1-12 G New : mylib/Process Noise I=1-12 G New  SystemSampleTime=-1  VariantActivationTime=update diagram  AllowFlexibleInterface=on  Latency=0  AutoFrameSizeCalculation=off
  XNSEG : Constant  Value=0.05
  XMNSEG : Outport  VectorParamsAs1DForOutWhenUnconnected=off
  G_NEW : Outport  Port=2  VectorParamsAs1DForOutWhenUnconnected=off
  wires:
  XNSEG/1 -> Process Noise I=1-12 G New/1
  Process Noise I=1-12 G New/1 -> XMNSEG/1
  G/1 -> Process Noise I=1-12 G New/2
  Process Noise I=1-12 G New/2 -> G_NEW/1

== system COSTEP_Exergy/Random number generator/Stream Measurements SMEAS Gas analysis1/If Action Subsystem3/Subsystem/Stream 3/Subsystem/TESUB6 XMNSEH ==
  G : Inport
  Process Noise I=1-12 G New : mylib/Process Noise I=1-12 G New  SystemSampleTime=-1  VariantActivationTime=update diagram  AllowFlexibleInterface=on  Latency=0  AutoFrameSizeCalculation=off
  XNSEH : Constant  Value=0.05
  XMNSEH : Outport  VectorParamsAs1DForOutWhenUnconnected=off
  G_NEW : Outport  Port=2  VectorParamsAs1DForOutWhenUnconnected=off
  wires:
  XNSEH/1 -> Process Noise I=1-12 G New/1
  Process Noise I=1-12 G New/1 -> XMNSEH/1
  G/1 -> Process Noise I=1-12 G New/2
  Process Noise I=1-12 G New/2 -> G_NEW/1

== system COSTEP_Exergy/Random number generator/Stream Measurements SMEAS Gas analysis1/If Action Subsystem3/Subsystem/Stream 4/Subsystem/TESUB6 XMNSEA ==
  G : Inport
  Process Noise I=1-12 G New : mylib/Process Noise I=1-12 G New  SystemSampleTime=-1  VariantActivationTime=update diagram  AllowFlexibleInterface=on  Latency=0  AutoFrameSizeCalculation=off
  XNSEA : Constant  Value=0.25
  XMNSEA : Outport  VectorParamsAs1DForOutWhenUnconnected=off
  G_NEW : Outport  Port=2  VectorParamsAs1DForOutWhenUnconnected=off
  wires:
  XNSEA/1 -> Process Noise I=1-12 G New/1
  Process Noise I=1-12 G New/1 -> XMNSEA/1
  G/1 -> Process Noise I=1-12 G New/2
  Process Noise I=1-12 G New/2 -> G_NEW/1

== system COSTEP_Exergy/Random number generator/Stream Measurements SMEAS Gas analysis1/If Action Subsystem3/Subsystem/Stream 4/Subsystem/TESUB6 XMNSEB ==
  G : Inport
  Process Noise I=1-12 G New : mylib/Process Noise I=1-12 G New  SystemSampleTime=-1  VariantActivationTime=update diagram  AllowFlexibleInterface=on  Latency=0  AutoFrameSizeCalculation=off
  XNSEB : Constant  Value=0.1
  XMNSEB : Outport  VectorParamsAs1DForOutWhenUnconnected=off
  G_NEW : Outport  Port=2  VectorParamsAs1DForOutWhenUnconnected=off
  wires:
  XNSEB/1 -> Process Noise I=1-12 G New/1
  Process Noise I=1-12 G New/1 -> XMNSEB/1
  G/1 -> Process Noise I=1-12 G New/2
  Process Noise I=1-12 G New/2 -> G_NEW/1

== system COSTEP_Exergy/Random number generator/Stream Measurements SMEAS Gas analysis1/If Action Subsystem3/Subsystem/Stream 4/Subsystem/TESUB6 XMNSEC ==
  G : Inport
  Process Noise I=1-12 G New : mylib/Process Noise I=1-12 G New  SystemSampleTime=-1  VariantActivationTime=update diagram  AllowFlexibleInterface=on  Latency=0  AutoFrameSizeCalculation=off
  XNSEC : Constant  Value=0.25
  XMNSEC : Outport  VectorParamsAs1DForOutWhenUnconnected=off
  G_NEW : Outport  Port=2  VectorParamsAs1DForOutWhenUnconnected=off
  wires:
  XNSEC/1 -> Process Noise I=1-12 G New/1
  Process Noise I=1-12 G New/1 -> XMNSEC/1
  G/1 -> Process Noise I=1-12 G New/2
  Process Noise I=1-12 G New/2 -> G_NEW/1

== system COSTEP_Exergy/Random number generator/Stream Measurements SMEAS Gas analysis1/If Action Subsystem3/Subsystem/Stream 4/Subsystem/TESUB6 XMNSED ==
  G : Inport
  Process Noise I=1-12 G New : mylib/Process Noise I=1-12 G New  SystemSampleTime=-1  VariantActivationTime=update diagram  AllowFlexibleInterface=on  Latency=0  AutoFrameSizeCalculation=off
  XNSED : Constant  Value=0.1
  XMNSED : Outport  VectorParamsAs1DForOutWhenUnconnected=off
  G_NEW : Outport  Port=2  VectorParamsAs1DForOutWhenUnconnected=off
  wires:
  XNSED/1 -> Process Noise I=1-12 G New/1
  Process Noise I=1-12 G New/1 -> XMNSED/1
  G/1 -> Process Noise I=1-12 G New/2
  Process Noise I=1-12 G New/2 -> G_NEW/1

== system COSTEP_Exergy/Random number generator/Stream Measurements SMEAS Gas analysis1/If Action Subsystem3/Subsystem/Stream 4/Subsystem/TESUB6 XMNSEE ==
  G : Inport
  Process Noise I=1-12 G New : mylib/Process Noise I=1-12 G New  SystemSampleTime=-1  VariantActivationTime=update diagram  AllowFlexibleInterface=on  Latency=0  AutoFrameSizeCalculation=off
  XNSEE : Constant  Value=0.25
  XMNSEE : Outport  VectorParamsAs1DForOutWhenUnconnected=off
  G_NEW : Outport  Port=2  VectorParamsAs1DForOutWhenUnconnected=off
  wires:
  XNSEE/1 -> Process Noise I=1-12 G New/1
  Process Noise I=1-12 G New/1 -> XMNSEE/1
  G/1 -> Process Noise I=1-12 G New/2
  Process Noise I=1-12 G New/2 -> G_NEW/1

== system COSTEP_Exergy/Random number generator/Stream Measurements SMEAS Gas analysis1/If Action Subsystem3/Subsystem/Stream 4/Subsystem/TESUB6 XMNSEF ==
  G : Inport
  Process Noise I=1-12 G New : mylib/Process Noise I=1-12 G New  SystemSampleTime=-1  VariantActivationTime=update diagram  AllowFlexibleInterface=on  Latency=0  AutoFrameSizeCalculation=off
  XNSEF : Constant  Value=0.025
  XMNSEF : Outport  VectorParamsAs1DForOutWhenUnconnected=off
  G_NEW : Outport  Port=2  VectorParamsAs1DForOutWhenUnconnected=off
  wires:
  XNSEF/1 -> Process Noise I=1-12 G New/1
  Process Noise I=1-12 G New/1 -> XMNSEF/1
  G/1 -> Process Noise I=1-12 G New/2
  Process Noise I=1-12 G New/2 -> G_NEW/1

== system COSTEP_Exergy/Random number generator/Stream Measurements SMEAS Gas analysis1/If Action Subsystem3/Subsystem/Stream 4/Subsystem/TESUB6 XMNSEG ==
  G : Inport
  Process Noise I=1-12 G New : mylib/Process Noise I=1-12 G New  SystemSampleTime=-1  VariantActivationTime=update diagram  AllowFlexibleInterface=on  Latency=0  AutoFrameSizeCalculation=off
  XNSEG : Constant  Value=0.05
  XMNSEG : Outport  VectorParamsAs1DForOutWhenUnconnected=off
  G_NEW : Outport  Port=2  VectorParamsAs1DForOutWhenUnconnected=off
  wires:
  XNSEG/1 -> Process Noise I=1-12 G New/1
  Process Noise I=1-12 G New/1 -> XMNSEG/1
  G/1 -> Process Noise I=1-12 G New/2
  Process Noise I=1-12 G New/2 -> G_NEW/1

== system COSTEP_Exergy/Random number generator/Stream Measurements SMEAS Gas analysis1/If Action Subsystem3/Subsystem/Stream 4/Subsystem/TESUB6 XMNSEH ==
  G : Inport
  Process Noise I=1-12 G New : mylib/Process Noise I=1-12 G New  SystemSampleTime=-1  VariantActivationTime=update diagram  AllowFlexibleInterface=on  Latency=0  AutoFrameSizeCalculation=off
  XNSEH : Constant  Value=0.05
  XMNSEH : Outport  VectorParamsAs1DForOutWhenUnconnected=off
  G_NEW : Outport  Port=2  VectorParamsAs1DForOutWhenUnconnected=off
  wires:
  XNSEH/1 -> Process Noise I=1-12 G New/1
  Process Noise I=1-12 G New/1 -> XMNSEH/1
  G/1 -> Process Noise I=1-12 G New/2
  Process Noise I=1-12 G New/2 -> G_NEW/1

== system COSTEP_Exergy/Random number generator/Stream Measurements SMEAS Gas analysis1/If Action Subsystem3/Subsystem/Stream 5/Subsystem/TESUB6 XMNSEA ==
  G : Inport
  Process Noise I=1-12 G New : mylib/Process Noise I=1-12 G New  SystemSampleTime=-1  VariantActivationTime=update diagram  AllowFlexibleInterface=on  Latency=0  AutoFrameSizeCalculation=off
  XNSEA : Constant  Value=0.25
  XMNSEA : Outport  VectorParamsAs1DForOutWhenUnconnected=off
  G_NEW : Outport  Port=2  VectorParamsAs1DForOutWhenUnconnected=off
  wires:
  XNSEA/1 -> Process Noise I=1-12 G New/1
  Process Noise I=1-12 G New/1 -> XMNSEA/1
  G/1 -> Process Noise I=1-12 G New/2
  Process Noise I=1-12 G New/2 -> G_NEW/1

== system COSTEP_Exergy/Random number generator/Stream Measurements SMEAS Gas analysis1/If Action Subsystem3/Subsystem/Stream 5/Subsystem/TESUB6 XMNSEB ==
  G : Inport
  Process Noise I=1-12 G New : mylib/Process Noise I=1-12 G New  SystemSampleTime=-1  VariantActivationTime=update diagram  AllowFlexibleInterface=on  Latency=0  AutoFrameSizeCalculation=off
  XNSEB : Constant  Value=0.1
  XMNSEB : Outport  VectorParamsAs1DForOutWhenUnconnected=off
  G_NEW : Outport  Port=2  VectorParamsAs1DForOutWhenUnconnected=off
  wires:
  XNSEB/1 -> Process Noise I=1-12 G New/1
  Process Noise I=1-12 G New/1 -> XMNSEB/1
  G/1 -> Process Noise I=1-12 G New/2
  Process Noise I=1-12 G New/2 -> G_NEW/1

== system COSTEP_Exergy/Random number generator/Stream Measurements SMEAS Gas analysis1/If Action Subsystem3/Subsystem/Stream 5/Subsystem/TESUB6 XMNSEC ==
  G : Inport
  Process Noise I=1-12 G New : mylib/Process Noise I=1-12 G New  SystemSampleTime=-1  VariantActivationTime=update diagram  AllowFlexibleInterface=on  Latency=0  AutoFrameSizeCalculation=off
  XNSEC : Constant  Value=0.25
  XMNSEC : Outport  VectorParamsAs1DForOutWhenUnconnected=off
  G_NEW : Outport  Port=2  VectorParamsAs1DForOutWhenUnconnected=off
  wires:
  XNSEC/1 -> Process Noise I=1-12 G New/1
  Process Noise I=1-12 G New/1 -> XMNSEC/1
  G/1 -> Process Noise I=1-12 G New/2
  Process Noise I=1-12 G New/2 -> G_NEW/1

== system COSTEP_Exergy/Random number generator/Stream Measurements SMEAS Gas analysis1/If Action Subsystem3/Subsystem/Stream 5/Subsystem/TESUB6 XMNSED ==
  G : Inport
  Process Noise I=1-12 G New : mylib/Process Noise I=1-12 G New  SystemSampleTime=-1  VariantActivationTime=update diagram  AllowFlexibleInterface=on  Latency=0  AutoFrameSizeCalculation=off
  XNSED : Constant  Value=0.1
  XMNSED : Outport  VectorParamsAs1DForOutWhenUnconnected=off
  G_NEW : Outport  Port=2  VectorParamsAs1DForOutWhenUnconnected=off
  wires:
  XNSED/1 -> Process Noise I=1-12 G New/1
  Process Noise I=1-12 G New/1 -> XMNSED/1
  G/1 -> Process Noise I=1-12 G New/2
  Process Noise I=1-12 G New/2 -> G_NEW/1
